simulink model "Boeing787_debug"  (R2013a)
settings: Solver=ode23tb  SolverMode=SingleTasking  StartTime=0.0  StopTime=18000  RelTol=1e-3
InitFcn:
  | load('SampleOutput.mat')
  | 
  | load('SampleFuelBurn.mat')
StartFcn:
  | tic
StopFcn:
  | ttt = toc
  | tend = eval(get_param(bdroot,'StopTime'));
  | disp(['Total Simulation Time (s) = ' num2str(ttt) 's']);
  | RTR =  ttt/tend
  | disp(['Simulation Speed is ' num2str(tend/ttt) 'x faster than real-time']);
values from neighbouring files (symbols this model uses):
  FuelBurn = [0 0 0 0 0 0 0 0 0 0 0 0 ... (18249 elements, 1x18249)]    [Benchmark_data1.mat]
undefined symbols (not defined in the file or in its folder): CurrentMission, seed
libraries: PowerFlowLib x20, simulink x14, powerlib_meascontrol x3
(part 15 of 17)

== system Boeing787_debug/Electrical/Generation Unit Sync-Sync5/Generator ==
  note: Dynamic model of P.U. Synchronous Generators v1.0
      | Base frequency is 60 Hz
      | Network transients are omitted
      | by Tutku Buyukdegirmenci
  note: Core Dynaimcs
  note: Outputs
  note: Inputs
  note: 0 axis to be implemented
  idq0 : Inport
  w : Inport  Port=2
  ifd' : Inport  Port=3
  Temp : Inport  Port=4
  Demux : Demux  Outputs=3
  Divide : Product  Inputs=*/
  Dynamics : Subsystem
  Electromagnetic Torque Output Power : Subsystem
  Gain1 : Gain  Gain=Xmd/R_fd/VBFD
  Gain2 : Gain  Gain=1/wB
  Gain3 : Gain  Gain=R_fd*VBFD/IBFD
  Gain4 : Gain  Gain=P/2
  Generator Power Loss : Subsystem
  Mux : Mux  Inputs=3
  Product : Product
  Stator Voltage : Subsystem
  Terminator2 : Terminator
  Terminator3 : Terminator
  Terminator4 : Terminator
  V0 : Constant  Value=0
  p.u. transform currents : Gain  Gain=-1/IBDQ
  p.u. transform torque : Gain  Gain=TB
  p.u. transform voltages : Gain  Gain=VBDQ
  vdq0 : Outport
  Te : Outport  Port=2
  vfd' : Outport  Port=3
  Ploss : Outport  Port=4
  wires:
  Gain4/1 -> Gain2/1
  [Efd] -> Dynamics/3(Efd)
  ifd'/1 -> Gain3/1
  idq0/1 -> p.u. transform currents/1
  p.u. transform voltages/1 -> vdq0/1
  Generator Power Loss/3(PLOSS) -> Ploss/1, Terminator4/1
  Generator Power Loss/2(PM) -> Terminator3/1
  Generator Power Loss/1(PE) -> Terminator2/1
  [Te] -> Generator Power Loss/5(Te)
  [nu] -> Generator Power Loss/6(w/ws)
  [Iq] -> Generator Power Loss/4(Iq)
  [Id] -> Generator Power Loss/3(Id)
  [Vq] -> Generator Power Loss/2(Eq)
  [Vd] -> Generator Power Loss/1(Ed)
  p.u. transform torque/1 -> Te/1
  p.u. transform currents/1 -> Demux/1
  [Te] -> p.u. transform torque/1
  Electromagnetic Torque Output Power/1(TE) -> [Te]
  [nu] -> Stator Voltage/7(w/ws)
  V0/1 -> Mux/3
  [Vq] -> Mux/2
  [Vd] -> Mux/1
  Mux/1 -> p.u. transform voltages/1
  [Iq] -> Electromagnetic Torque Output Power/2(Iq), Stator Voltage/2(Iq)
  [Id] -> Electromagnetic Torque Output Power/1(Id), Stator Voltage/1(Id)
  [Iq] -> Dynamics/2(Iq)
  [Id] -> Dynamics/1(Id)
  Gain2/1 -> [nu]
  Demux/2 -> [Iq]
  Demux/1 -> [Id]
  w/1 -> Gain4/1
  Stator Voltage/1(Ed) -> [Vd]
  Stator Voltage/2(Eq) -> [Vq]
  Dynamics/4(Phi_2q) -> Electromagnetic Torque Output Power/6(Phi_2q), Stator Voltage/6(Phi_2q)
  Dynamics/3(Phi_1d) -> Electromagnetic Torque Output Power/5(Phi_1d), Stator Voltage/5(Phi_1d)
  Dynamics/2(Ed1) -> Electromagnetic Torque Output Power/4(Ed1), Stator Voltage/4(Ed1)
  Dynamics/1(Eq1) -> Electromagnetic Torque Output Power/3(Eq1), Stator Voltage/3(Eq1)
  Temp/1 -> [R_temp_delta]
  Gain1/1 -> Divide/1
  Divide/1 -> [Efd]
  Gain3/1 -> Product/1  "vfd'"
  Product/1 -> Gain1/1, vfd'/1
  [R_temp_delta] -> Divide/2, Product/2
  [R_temp_delta] -> Stator Voltage/8(Temp), Dynamics/4(Temp)

== system Boeing787_debug/Electrical/Thermal Interface/Battery Thermal Model ==
  Ploss : Inport
  Liquid Coolant Temp : Inport  Port=2
  Air Temp : Inport  Port=3
  coolant mdot : Inport  Port=4
  Integrator : Integrator  InitialCondition=20
  MATLAB Function : MATLAB Function  TreatAsAtomicUnit=on
  T_Batt : Outport
  wires:
  Ploss/1 -> MATLAB Function/1(Ploss)
  Liquid Coolant Temp/1 -> MATLAB Function/2(Tf)
  MATLAB Function/1(Tdot) -> Integrator/1
  Integrator/1 -> MATLAB Function/5(Tgen), T_Batt/1
  coolant mdot/1 -> MATLAB Function/4(mdot_f)
  Air Temp/1 -> MATLAB Function/3(Ta)

== system Boeing787_debug/Electrical/Thermal Interface/Generator 1 Thermal Model ==
  Ploss : Inport
  Liquid Coolant Temp : Inport  Port=2
  Air Temp : Inport  Port=3
  coolant mdot : Inport  Port=4
  Integrator : Integrator  InitialCondition=20
  MATLAB Function : MATLAB Function  TreatAsAtomicUnit=on
  T_gen : Outport
  wires:
  Ploss/1 -> MATLAB Function/1(Ploss)
  Liquid Coolant Temp/1 -> MATLAB Function/2(Tf)
  MATLAB Function/1(Tdot) -> Integrator/1
  Integrator/1 -> MATLAB Function/5(Tgen), T_gen/1
  coolant mdot/1 -> MATLAB Function/4(mdot_f)
  Air Temp/1 -> MATLAB Function/3(Ta)

== system Boeing787_debug/Electrical/Thermal Interface/Generator 2 Thermal Model ==
  Ploss : Inport
  Liquid Coolant Temp : Inport  Port=2
  Air Temp : Inport  Port=3
  coolant mdot : Inport  Port=4
  Integrator : Integrator  InitialCondition=20
  MATLAB Function : MATLAB Function  TreatAsAtomicUnit=on
  T_gen : Outport
  wires:
  Air Temp/1 -> MATLAB Function/3(Ta)
  coolant mdot/1 -> MATLAB Function/4(mdot_f)
  Integrator/1 -> T_gen/1, MATLAB Function/5(Tgen)
  MATLAB Function/1(Tdot) -> Integrator/1
  Liquid Coolant Temp/1 -> MATLAB Function/2(Tf)
  Ploss/1 -> MATLAB Function/1(Ploss)

== system Boeing787_debug/Electrical/Thermal Interface/Generator 3 Thermal Model ==
  Ploss : Inport
  Liquid Coolant Temp : Inport  Port=2
  Air Temp : Inport  Port=3
  coolant mdot : Inport  Port=4
  Integrator : Integrator  InitialCondition=20
  MATLAB Function : MATLAB Function  TreatAsAtomicUnit=on
  T_gen : Outport
  wires:
  Ploss/1 -> MATLAB Function/1(Ploss)
  Liquid Coolant Temp/1 -> MATLAB Function/2(Tf)
  MATLAB Function/1(Tdot) -> Integrator/1
  Integrator/1 -> MATLAB Function/5(Tgen), T_gen/1
  coolant mdot/1 -> MATLAB Function/4(mdot_f)
  Air Temp/1 -> MATLAB Function/3(Ta)

== system Boeing787_debug/Electrical/Thermal Interface/Generator 4 Thermal Model ==
  Ploss : Inport
  Liquid Coolant Temp : Inport  Port=2
  Air Temp : Inport  Port=3
  coolant mdot : Inport  Port=4
  Integrator : Integrator  InitialCondition=20
  MATLAB Function : MATLAB Function  TreatAsAtomicUnit=on
  T_gen : Outport
  wires:
  Air Temp/1 -> MATLAB Function/3(Ta)
  coolant mdot/1 -> MATLAB Function/4(mdot_f)
  Integrator/1 -> T_gen/1, MATLAB Function/5(Tgen)
  MATLAB Function/1(Tdot) -> Integrator/1
  Liquid Coolant Temp/1 -> MATLAB Function/2(Tf)
  Ploss/1 -> MATLAB Function/1(Ploss)

== system Boeing787_debug/Electrical/Thermal Interface/Generator 5 Thermal Model ==
  Ploss : Inport
  Liquid Coolant Temp : Inport  Port=2
  Air Temp : Inport  Port=3
  coolant mdot : Inport  Port=4
  Integrator : Integrator  InitialCondition=20
  MATLAB Function : MATLAB Function  TreatAsAtomicUnit=on
  T_gen : Outport
  wires:
  Ploss/1 -> MATLAB Function/1(Ploss)
  Liquid Coolant Temp/1 -> MATLAB Function/2(Tf)
  MATLAB Function/1(Tdot) -> Integrator/1
  Integrator/1 -> MATLAB Function/5(Tgen), T_gen/1
  coolant mdot/1 -> MATLAB Function/4(mdot_f)
  Air Temp/1 -> MATLAB Function/3(Ta)

== system Boeing787_debug/Electrical/Thermal Interface/Generator 6 Thermal Model ==
  Ploss : Inport
  Liquid Coolant Temp : Inport  Port=2
  Air Temp : Inport  Port=3
  coolant mdot : Inport  Port=4
  Integrator : Integrator  InitialCondition=20
  MATLAB Function : MATLAB Function  TreatAsAtomicUnit=on
  T_gen : Outport
  wires:
  Air Temp/1 -> MATLAB Function/3(Ta)
  coolant mdot/1 -> MATLAB Function/4(mdot_f)
  Integrator/1 -> T_gen/1, MATLAB Function/5(Tgen)
  MATLAB Function/1(Tdot) -> Integrator/1
  Liquid Coolant Temp/1 -> MATLAB Function/2(Tf)
  Ploss/1 -> MATLAB Function/1(Ploss)

== system Boeing787_debug/Electrical/Thermal Interface/Load Thermal Model ==
  Ploss : Inport
  Liquid Coolant Temp : Inport  Port=2
  Air Temp : Inport  Port=3
  coolant mdot : Inport  Port=4
  Integrator : Integrator  InitialCondition=20
  MATLAB Function : MATLAB Function  TreatAsAtomicUnit=on
  T_gen : Outport
  wires:
  Air Temp/1 -> MATLAB Function/3(Ta)
  coolant mdot/1 -> MATLAB Function/4(mdot_f)
  Integrator/1 -> T_gen/1, MATLAB Function/5(Tgen)
  MATLAB Function/1(Tdot) -> Integrator/1
  Liquid Coolant Temp/1 -> MATLAB Function/2(Tf)
  Ploss/1 -> MATLAB Function/1(Ploss)

== system Boeing787_debug/Electrical/Transformer-rectifier/Control New ==
  Vout : Inport
  ref : Inport  Port=2
  Gain1 : Gain
  Integrator1 : Integrator  ExternalReset=rising
  Ki1 : Gain  Gain=10
  Kp e(t)1 : Gain  Gain=10
  PID Controller : simulink/Continuous/PID Controller  Controller=PID  TimeDomain=Continuous-time  SampleTime=1  IntegratorMethod=Forward Euler  FilterMethod=Forward Euler  Form=Parallel  P=0  I=-20.0000452359282  D=0  N=100  InitialConditionSource=internal  InitialConditionForIntegrator=0  InitialConditionForFilter=0  ExternalReset=none  LimitOutput=off  UpperSaturationLimit=inf  LowerSaturationLimit=-inf  LinearizeAsGain=on  AntiWindupMode=none  Kb=1  TrackingMode=off  Kt=1  PParamMin=[]  PParamMax=[]  IParamMin=[]  IParamMax=[]  DParamMin=[]  DParamMax=[]  NParamMin=[]  NParamMax=[]  KbParamMin=[]  KbParamMax=[]  KtParamMin=[]  KtParamMax=[]  POutMin=[]  POutMax=[]  IOutMin=[]  IOutMax=[]  DOutMin=[]  DOutMax=[]  NOutMin=[]  NOutMax=[]  KbOutMin=[]  KbOutMax=[]  KtOutMin=[]  KtOutMax=[]  IntegratorOutMin=[]  IntegratorOutMax=[]  FilterOutMin=[]  FilterOutMax=[]  SumOutMin=[]  SumOutMax=[]  SumI1OutMin=[]  SumI1OutMax=[]  SumI2OutMin=[]  SumI2OutMax=[]  SumI3OutMin=[]  SumI3OutMax=[]  SumDOutMin=[]  SumDOutMax=[]  SaturationOutMin=[]  SaturationOutMax=[]  IntegratorContinuousStateAttributes=''  IntegratorStateMustResolveToSignalObject=off  IntegratorRTWStateStorageClass=Auto  FilterContinuousStateAttributes=''  FilterStateMustResolveToSignalObject=off  FilterRTWStateStorageClass=Auto
  Reset on controller start1 : Step  Time=75  SampleTime=0
  Sum : Sum  Inputs=|-+
  Sum2 : Sum  Inputs=|++
  u : Outport
  wires:
  Sum/1 -> PID Controller/1
  Integrator1/1 -> Sum2/1
  Kp e(t)1/1 -> Sum2/2
  Ki1/1 -> Integrator1/1
  Reset on controller start1/1 -> Integrator1/2
  ? -> Kp e(t)1/1, Ki1/1
  Gain1/1 -> u/1
  ref/1 -> Sum/2
  Vout/1 -> Sum/1
  PID Controller/1 -> Gain1/1

== system Boeing787_debug/Electrical/Transformer-rectifier/Control old ==
  Vout : Inport
  ref : Inport  Port=2
  Clock : Clock
  Constant2 : Constant  Value=0
  Dead Zone : DeadZone  LowerValue=-2  UpperValue=2  SaturateOnIntegerOverflow=on
  Gain : Gain
  Gain1 : Gain  Gain=-1
  Integrator : Integrator  ExternalReset=rising
  MinMax : MinMax  Function=max
  Reset on controller start : Step  Time=75  SampleTime=0
  Sum : Sum  Inputs=|-+
  Switch : Switch  Criteria=u2 > Threshold  Threshold=75
  u : Outport
  wires:
  Vout/1 -> MinMax/1
  Dead Zone/1 -> Gain/1
  Gain1/1 -> u/1
  Gain/1 -> Integrator/1
  ref/1 -> Sum/2
  Clock/1 -> Switch/2
  Constant2/1 -> Switch/3
  MinMax/1 -> Sum/1
  Switch/1 -> Gain1/1
  Reset on controller start/1 -> Integrator/2
  Sum/1 -> Dead Zone/1
  Integrator/1 -> Switch/1

== system Boeing787_debug/Electrical/Transformer-rectifier/Three-phase Full Bridge Rectifier ==
  iout : Inport
  vin : Inport  Port=2
  u : Inport  Port=3
  1/C : Gain  Gain=1/C  SaturateOnIntegerOverflow=on  OutDataTypeStr=Inherit: Same as input  ParamDataTypeStr=Inherit: Same as input
  1/Rc : Gain  Gain=1/Rc  SaturateOnIntegerOverflow=on  OutDataTypeStr=Inherit: Same as input  ParamDataTypeStr=Inherit: Same as input
  Abs : Abs  SaturateOnIntegerOverflow=on
  Constant : Constant
  Constant1 : Constant  Value=800*pi
  Demux : Demux  Outputs=3
  Demux1 : Demux  Outputs=3
  Integrator : Integrator
  MinMax1 : MinMax  Function=max
  Mux : Mux  Inputs=3
  Mux1 : Mux  Inputs=3
  Product : Product  RndMeth=Zero
  Saturation : Saturate  UpperLimit=inf  LowerLimit=0
  Sum{,1..7} (8 alike) : Sum  Inputs=+-  SaturateOnIntegerOverflow=on  InputSameDT=on  OutDataTypeStr=Inherit: Same as first input
  Sum8 : Sum  Inputs=|++
  dq0 to abc : powerlib_meascontrol/Transformations/dq0 to abc  Alignment=90 degrees behind phase A axis
  vout : Outport
  iin : Outport  Port=2
  wires:
  Saturation/1 -> Sum1/1, Product/2
  1/C/1 -> Integrator/1
  Sum1/1 -> 1/C/1
  Integrator/1 -> Sum8/1, vout/1
  1/Rc/1 -> Saturation/1
  iout/1 -> Sum1/2
  Sum/1 -> 1/Rc/1
  Product/1 -> iin/1
  MinMax1/1 -> Sum/1
  Abs/1 -> MinMax1/1
  u/1 -> Sum8/2
  Sum8/1 -> Sum/2
  Constant/1 -> Product/1
  ? -> Demux1/1
  Mux1/1 -> ?
  Demux1/1 -> Sum7/2, Sum5/1
  Demux1/2 -> Sum5/2, Sum6/1
  Demux1/3 -> Sum7/1, Sum6/2
  Sum5/1 -> Mux1/1
  Sum6/1 -> Mux1/2
  Sum7/1 -> Mux1/3
  Sum4/1 -> Mux/3
  Sum3/1 -> Mux/2
  Sum2/1 -> Mux/1
  Demux/3 -> Sum3/2, Sum4/1
  Demux/2 -> Sum3/1, Sum2/2
  Demux/1 -> Sum2/1, Sum4/2
  Mux/1 -> Abs/1
  vin/1 -> dq0 to abc/1
  dq0 to abc/1 -> Demux/1
  Constant1/1 -> dq0 to abc/2

== system Boeing787_debug/Electrical/Transformer-rectifier/Transformer1 ==
  Vin : Inport
  Iout : Inport  Port=2
  Gain : Gain  Gain=N2/N1
  Gain1 : Gain  Gain=N2/N1
  Gain2 : Gain  Gain=Rp
  Gain3 : Gain  Gain=Rs
  Scope : Scope
      settings: YMin=-28.76938  YMax=258.92445  SaveName=ScopeData11
  Sum1 : Sum  Inputs=|+-
  Sum2 : Sum  Inputs=|+-
  Vout : Outport
  Iin : Outport  Port=2
  wires:
  Gain3/1 -> Sum2/2
  Gain1/1 -> Iin/1, Gain2/1
  Sum2/1 -> Vout/1
  Gain/1 -> Sum2/1
  Sum1/1 -> Gain/1
  Gain2/1 -> Sum1/2
  Vin/1 -> Sum1/1
  Iout/1 -> Scope/1, Gain3/1, Gain1/1

== system Boeing787_debug/Electrical/Transformer-rectifier1/Control New ==
  Vout : Inport
  ref : Inport  Port=2
  Gain1 : Gain
  Integrator1 : Integrator  ExternalReset=rising
  Ki1 : Gain  Gain=10
  Kp e(t)1 : Gain  Gain=10
  PID Controller : simulink/Continuous/PID Controller  Controller=PID  TimeDomain=Continuous-time  SampleTime=1  IntegratorMethod=Forward Euler  FilterMethod=Forward Euler  Form=Parallel  P=0  I=-20.0000452359282  D=0  N=100  InitialConditionSource=internal  InitialConditionForIntegrator=0  InitialConditionForFilter=0  ExternalReset=none  LimitOutput=off  UpperSaturationLimit=inf  LowerSaturationLimit=-inf  LinearizeAsGain=on  AntiWindupMode=none  Kb=1  TrackingMode=off  Kt=1  PParamMin=[]  PParamMax=[]  IParamMin=[]  IParamMax=[]  DParamMin=[]  DParamMax=[]  NParamMin=[]  NParamMax=[]  KbParamMin=[]  KbParamMax=[]  KtParamMin=[]  KtParamMax=[]  POutMin=[]  POutMax=[]  IOutMin=[]  IOutMax=[]  DOutMin=[]  DOutMax=[]  NOutMin=[]  NOutMax=[]  KbOutMin=[]  KbOutMax=[]  KtOutMin=[]  KtOutMax=[]  IntegratorOutMin=[]  IntegratorOutMax=[]  FilterOutMin=[]  FilterOutMax=[]  SumOutMin=[]  SumOutMax=[]  SumI1OutMin=[]  SumI1OutMax=[]  SumI2OutMin=[]  SumI2OutMax=[]  SumI3OutMin=[]  SumI3OutMax=[]  SumDOutMin=[]  SumDOutMax=[]  SaturationOutMin=[]  SaturationOutMax=[]  IntegratorContinuousStateAttributes=''  IntegratorStateMustResolveToSignalObject=off  IntegratorRTWStateStorageClass=Auto  FilterContinuousStateAttributes=''  FilterStateMustResolveToSignalObject=off  FilterRTWStateStorageClass=Auto
  Reset on controller start1 : Step  Time=75  SampleTime=0
  Sum : Sum  Inputs=|-+
  Sum2 : Sum  Inputs=|++
  u : Outport
  wires:
  Sum/1 -> PID Controller/1
  Integrator1/1 -> Sum2/1
  Kp e(t)1/1 -> Sum2/2
  Ki1/1 -> Integrator1/1
  Reset on controller start1/1 -> Integrator1/2
  ? -> Kp e(t)1/1, Ki1/1
  Gain1/1 -> u/1
  ref/1 -> Sum/2
  Vout/1 -> Sum/1
  PID Controller/1 -> Gain1/1

== system Boeing787_debug/Electrical/Transformer-rectifier1/Control old ==
  Vout : Inport
  ref : Inport  Port=2
  Clock : Clock
  Constant2 : Constant  Value=0
  Gain1 : Gain  Gain=-1
  Integrator : Integrator  ExternalReset=rising
  Ki : Gain  Gain=10
  Kp e(t) : Gain  Gain=10
  MinMax : MinMax  Function=max
  Reset on controller start : Step  Time=75  SampleTime=0
  Sum : Sum  Inputs=|-+
  Sum1 : Sum  Inputs=|++
  Switch : Switch  Criteria=u2 > Threshold  Threshold=75
  u : Outport
  wires:
  Vout/1 -> MinMax/1
  Sum/1 -> Kp e(t)/1, Ki/1
  Reset on controller start/1 -> Integrator/2
  Switch/1 -> Gain1/1
  MinMax/1 -> Sum/1
  Constant2/1 -> Switch/3
  Clock/1 -> Switch/2
  ref/1 -> Sum/2
  Ki/1 -> Integrator/1
  Gain1/1 -> u/1
  Kp e(t)/1 -> Sum1/2
  Integrator/1 -> Sum1/1
  Sum1/1 -> Switch/1

== system Boeing787_debug/Electrical/Transformer-rectifier1/Three-phase Full Bridge1 ==
  iout : Inport
  vin : Inport  Port=2
  u : Inport  Port=3
  vin1 : Inport  Port=4
  1/C : Gain  Gain=1/C  SaturateOnIntegerOverflow=on  OutDataTypeStr=Inherit: Same as input  ParamDataTypeStr=Inherit: Same as input
  1/Rc : Gain  Gain=1/Rc  SaturateOnIntegerOverflow=on  OutDataTypeStr=Inherit: Same as input  ParamDataTypeStr=Inherit: Same as input
  Abs : Abs  SaturateOnIntegerOverflow=on
  Constant : Constant  Value=800*pi
  Demux : Demux  Outputs=3
  Demux1 : Demux  Outputs=3
  Integrator : Integrator
  MinMax1 : MinMax  Function=max
  Mux : Mux  Inputs=3
  Mux1 : Mux  Inputs=3
  Saturation : Saturate  UpperLimit=inf  LowerLimit=0
  Scope : Scope
      settings: YMin=-3.32249  YMax=29.90241  SaveName=ScopeData12
  Sum{,1..4,6..8} (8 alike) : Sum  Inputs=+-  SaturateOnIntegerOverflow=on  InputSameDT=on  OutDataTypeStr=Inherit: Same as first input
  Sum5 : Sum  SaturateOnIntegerOverflow=on  InputSameDT=on  OutDataTypeStr=Inherit: Same as first input
  dq0 to abc : powerlib_meascontrol/Transformations/dq0 to abc  Alignment=90 degrees behind phase A axis
  vout : Outport
  iin : Outport  Port=2
  wires:
  Sum5/1 -> Sum/2
  u/1 -> Sum5/2
  Abs/1 -> MinMax1/1
  MinMax1/1 -> Sum/1
  Saturation/1 -> iin/1, Scope/1, Sum1/1
  Sum/1 -> 1/Rc/1
  iout/1 -> Sum1/2
  1/Rc/1 -> Saturation/1
  Integrator/1 -> Sum5/1, vout/1
  Sum1/1 -> 1/C/1
  1/C/1 -> Integrator/1
  Sum8/1 -> Mux1/3
  Sum7/1 -> Mux1/2
  Sum6/1 -> Mux1/1
  Demux1/3 -> Sum7/2, Sum8/1
  Demux1/2 -> Sum7/1, Sum6/2
  Demux1/1 -> Sum6/1, Sum8/2
  Mux1/1 -> ?
  vin1/1 -> Demux1/1
  Sum4/1 -> Mux/3
  Sum3/1 -> Mux/2
  Sum2/1 -> Mux/1
  Demux/3 -> Sum3/2, Sum4/1
  Demux/2 -> Sum3/1, Sum2/2
  Demux/1 -> Sum2/1, Sum4/2
  Mux/1 -> Abs/1
  dq0 to abc/1 -> Demux/1
  vin/1 -> dq0 to abc/1
  Constant/1 -> dq0 to abc/2

== system Boeing787_debug/Electrical/Transformer-rectifier1/Transformer1 ==
  Vin : Inport
  Iout : Inport  Port=2
  Gain : Gain  Gain=N2/N1
  Gain1 : Gain  Gain=N2/N1
  Gain2 : Gain  Gain=Rp
  Gain3 : Gain  Gain=Rs
  Memory1 : Memory
  Scope : Scope
      settings: YMin=-1.03024  YMax=9.27213  SaveName=ScopeData11
  Sum1 : Sum  Inputs=|+-
  Sum2 : Sum  Inputs=|+-
  Vout : Outport
  Iin : Outport  Port=2
  wires:
  Memory1/1 -> Gain1/1, Gain3/1, Scope/1
  Iout/1 -> Memory1/1
  Vin/1 -> Sum1/1
  Gain2/1 -> Sum1/2
  Sum1/1 -> Gain/1
  Gain/1 -> Sum2/1
  Sum2/1 -> Vout/1
  Gain1/1 -> Gain2/1, Iin/1
  Gain3/1 -> Sum2/2

== system Boeing787_debug/Electrical/Enabled_AC_Loadloss/Enabled Subsystem/CURRENT BASED LOADS ==
  note: SPLITTING CURRENT IN BOTH D AND Q AXES
  Constant : Constant  Value=0
  Constant1 : Constant  Value=ILRMS
  Gain1 : Gain  Gain=sqrt(2)
  Mux : Mux  Inputs=3
  Idqo : Outport
  wires:
  Constant/1 -> Mux/3
  Mux/1 -> Idqo/1
  Gain1/1 -> Mux/2, Mux/1
  Constant1/1 -> Gain1/1

== system Boeing787_debug/Electrical/Enabled_AC_Loadloss/Enabled Subsystem/IMPEDANCE BASED LOADS ==
  Vdq0 : Inport
  Constant1 : Constant  Value=R
  Constant2 : Constant  Value=X
  Constant3 : Constant  Value=R
  Constant4 : Constant  Value=X
  Demux : Demux  Outputs=3
  Fcn : Fcn  Expr=u(1)/(u(2)+0.1)
  Fcn1 : Fcn  Expr=u(1)/(u(2)+0.1)
  Math Function{,1..3} (4 alike) : Math  Operator=square  SaturateOnIntegerOverflow=on
  Mux : Mux  Inputs=3
  Mux1 : Mux  Inputs=2
  Mux2 : Mux  Inputs=2
  Product{1..2,5..6} (4 alike) : Product  Inputs=**  RndMeth=Zero
  Sum1 : Sum  Inputs=|++
  Sum2 : Sum  Inputs=|++
  Sum3 : Sum  Inputs=|+-
  Sum4 : Sum  Inputs=|++
  Idq0 : Outport
  wires:
  Fcn1/1 -> Mux/2
  Fcn/1 -> Mux/1
  Vdq0/1 -> Demux/1
  Constant1/1 -> Product1/1, Math Function/1
  Demux/1 -> Product1/2, Product6/2
  Product1/1 -> Sum1/1
  Demux/2 -> Product2/2, Product5/2
  Constant2/1 -> Product2/1, Math Function1/1
  Product2/1 -> Sum1/2
  Sum1/1 -> Mux1/1
  Math Function/1 -> Sum2/1
  Math Function1/1 -> Sum2/2
  Sum2/1 -> Mux1/2
  Constant3/1 -> Product5/1, Math Function2/1
  Product5/1 -> Sum3/1
  Constant4/1 -> Product6/1, Math Function3/1
  Product6/1 -> Sum3/2
  Math Function2/1 -> Sum4/1
  Math Function3/1 -> Sum4/2
  Sum3/1 -> Mux2/1
  Sum4/1 -> Mux2/2
  Mux1/1 -> Fcn/1
  Mux2/1 -> Fcn1/1
  Mux/1 -> Idq0/1

== system Boeing787_debug/Electrical/Enabled_AC_Loadloss/Enabled Subsystem/POWER BASED LOADS ==
  Vdq0 : Inport
  Constant1 : Constant  Value=P
  Constant2 : Constant  Value=PF
  Constant3 : Constant  Value=P
  Constant5 : Constant
  Constant6 : Constant  Value=0
  Constant7 : Constant  Value=P
  Demux : Demux  Outputs=3
  Fcn : Fcn  Expr=u(1)/(u(2)+0.1)
  Fcn1 : Fcn  Expr=u(1)/(u(2)+0.1)
  Math Function{,1..3} (4 alike) : Math  Operator=square  SaturateOnIntegerOverflow=on
  Mux : Mux  Inputs=3
  Mux1 : Mux  Inputs=2
  Mux2 : Mux  Inputs=2
  Product1 : Product  Inputs=***  RndMeth=Zero
  Product2 : Product  Inputs=**  RndMeth=Zero
  Product3 : Product  Inputs=**  RndMeth=Zero
  Product5 : Product  Inputs=***  RndMeth=Zero
  Product6 : Product  Inputs=**  RndMeth=Zero
  Sum1 : Sum  Inputs=|++
  Sum2 : Sum  Inputs=|++
  Sum3 : Sum  Inputs=|+-
  Sum4 : Sum  Inputs=|++
  Trigonometric Function : Trigonometry  Operator=acos
  Trigonometric Function1 : Trigonometry  Operator=tan
  Idq0 : Outport
  loss : Outport  Port=2
  wires:
  Constant1/1 -> Product1/1, loss/1
  Constant6/1 -> Product5/3
  Constant5/1 -> Product1/3
  Mux/1 -> Idq0/1
  Mux2/1 -> Fcn1/1
  Mux1/1 -> Fcn/1
  Sum4/1 -> Mux2/2
  Sum3/1 -> Mux2/1
  Math Function3/1 -> Sum4/2
  Math Function2/1 -> Sum4/1
  Product6/1 -> Sum3/2
  Product3/1 -> Product6/1, Product2/1
  Product5/1 -> Sum3/1
  Constant3/1 -> Product5/1
  Sum2/1 -> Mux1/2
  Math Function1/1 -> Sum2/2
  Math Function/1 -> Sum2/1
  Sum1/1 -> Mux1/1
  Product2/1 -> Sum1/2
  Constant2/1 -> Trigonometric Function/1
  Demux/2 -> Math Function2/1, Product5/2, Math Function1/1, Product2/2
  Product1/1 -> Sum1/1
  Demux/1 -> Math Function3/1, Product6/2, Math Function/1, Product1/2
  Vdq0/1 -> Demux/1
  Fcn/1 -> Mux/1
  Fcn1/1 -> Mux/2
  Trigonometric Function/1 -> Trigonometric Function1/1
  Trigonometric Function1/1 -> Product3/1
  Constant7/1 -> Product3/2

== system Boeing787_debug/Electrical/Enabled_AC_Loadloss/Enabled Subsystem1/CURRENT BASED LOADS ==
  note: SPLITTING CURRENT IN BOTH D AND Q AXES
  Iconst RMS : Inport
  Gain1 : Gain  Gain=sqrt(2)
  Mux : Mux  Inputs=3
  Idqo : Outport
  wires:
  Iconst RMS/1 -> Gain1/1
  Gain1/1 -> Mux/1, Mux/2
  Mux/1 -> Idqo/1

== system Boeing787_debug/Electrical/Enabled_AC_Loadloss/Enabled Subsystem1/POWER BASED LOADS ==
  Vdq0 : Inport
  P : Inport  Port=2
  Q : Inport  Port=3
  Demux : Demux  Outputs=3
  Fcn : Fcn  Expr=u(1)/(u(2)+0.1)
  Fcn1 : Fcn  Expr=u(1)/(u(2)+0.1)
  Math Function{,1..3} (4 alike) : Math  Operator=square  SaturateOnIntegerOverflow=on
  Mux : Mux  Inputs=3
  Mux1 : Mux  Inputs=2
  Mux2 : Mux  Inputs=2
  Product{1..2,5..6} (4 alike) : Product  Inputs=**  RndMeth=Zero
  Sum1 : Sum  Inputs=|++
  Sum2 : Sum  Inputs=|++
  Sum3 : Sum  Inputs=|+-
  Sum4 : Sum  Inputs=|++
  Idq0 : Outport
  wires:
  Demux/1 -> Math Function/1, Product1/2, Product6/2, Math Function3/1
  Vdq0/1 -> Demux/1
  P/1 -> Product1/1, Product5/1
  Product1/1 -> Sum1/1
  Demux/2 -> Product2/2, Math Function1/1, Product5/2, Math Function2/1
  Q/1 -> Product2/1, Product6/1
  Product2/1 -> Sum1/2
  Sum1/1 -> Mux1/1
  Math Function/1 -> Sum2/1
  Math Function1/1 -> Sum2/2
  Sum2/1 -> Mux1/2
  Product5/1 -> Sum3/1
  Product6/1 -> Sum3/2
  Math Function2/1 -> Sum4/1
  Math Function3/1 -> Sum4/2
  Sum3/1 -> Mux2/1
  Sum4/1 -> Mux2/2
  Mux1/1 -> Fcn/1
  Mux2/1 -> Fcn1/1
  Mux/1 -> Idq0/1
  Fcn/1 -> Mux/1
  Fcn1/1 -> Mux/2

== system Boeing787_debug/Electrical/Enabled_AC_Loadloss1/Enabled Subsystem/CURRENT BASED LOADS ==
  note: SPLITTING CURRENT IN BOTH D AND Q AXES
  Constant : Constant  Value=0
  Constant1 : Constant  Value=ILRMS
  Gain1 : Gain  Gain=sqrt(2)
  Mux : Mux  Inputs=3
  Idqo : Outport
  wires:
  Constant/1 -> Mux/3
  Mux/1 -> Idqo/1
  Gain1/1 -> Mux/2, Mux/1
  Constant1/1 -> Gain1/1

== system Boeing787_debug/Electrical/Enabled_AC_Loadloss1/Enabled Subsystem/IMPEDANCE BASED LOADS ==
  Vdq0 : Inport
  Constant1 : Constant  Value=R
  Constant2 : Constant  Value=X
  Constant3 : Constant  Value=R
  Constant4 : Constant  Value=X
  Demux : Demux  Outputs=3
  Fcn : Fcn  Expr=u(1)/(u(2)+0.1)
  Fcn1 : Fcn  Expr=u(1)/(u(2)+0.1)
  Math Function{,1..3} (4 alike) : Math  Operator=square  SaturateOnIntegerOverflow=on
  Mux : Mux  Inputs=3
  Mux1 : Mux  Inputs=2
  Mux2 : Mux  Inputs=2
  Product{1..2,5..6} (4 alike) : Product  Inputs=**  RndMeth=Zero
  Sum1 : Sum  Inputs=|++
  Sum2 : Sum  Inputs=|++
  Sum3 : Sum  Inputs=|+-
  Sum4 : Sum  Inputs=|++
  Transfer Fcn1 : TransferFcn  Denominator=[.01 1]
  Transfer Fcn2 : TransferFcn  Denominator=[.01 1]
  Idq0 : Outport
  wires:
  Fcn1/1 -> Transfer Fcn1/1
  Fcn/1 -> Transfer Fcn2/1
  Vdq0/1 -> Demux/1
  Constant1/1 -> Product1/1, Math Function/1
  Demux/1 -> Product1/2, Product6/2
  Product1/1 -> Sum1/1
  Demux/2 -> Product2/2, Product5/2
  Constant2/1 -> Product2/1, Math Function1/1
  Product2/1 -> Sum1/2
  Sum1/1 -> Mux1/1
  Math Function/1 -> Sum2/1
  Math Function1/1 -> Sum2/2
  Sum2/1 -> Mux1/2
  Constant3/1 -> Product5/1, Math Function2/1
  Product5/1 -> Sum3/1
  Constant4/1 -> Product6/1, Math Function3/1
  Product6/1 -> Sum3/2
  Math Function2/1 -> Sum4/1
  Math Function3/1 -> Sum4/2
  Sum3/1 -> Mux2/1
  Sum4/1 -> Mux2/2
  Mux1/1 -> Fcn/1
  Mux2/1 -> Fcn1/1
  Mux/1 -> Idq0/1
  Transfer Fcn2/1 -> Mux/1
  Transfer Fcn1/1 -> Mux/2

== system Boeing787_debug/Electrical/Enabled_AC_Loadloss1/Enabled Subsystem/POWER BASED LOADS ==
  Vdq0 : Inport
  Constant1 : Constant  Value=P
  Constant2 : Constant  Value=PF
  Constant3 : Constant  Value=P
  Constant5 : Constant
  Constant6 : Constant  Value=0
  Constant7 : Constant  Value=P
  Demux : Demux  Outputs=3
  Fcn : Fcn  Expr=u(1)/(u(2)+0.1)
  Fcn1 : Fcn  Expr=u(1)/(u(2)+0.1)
  Math Function{,1..3} (4 alike) : Math  Operator=square  SaturateOnIntegerOverflow=on
  Mux : Mux  Inputs=3
  Mux1 : Mux  Inputs=2
  Mux2 : Mux  Inputs=2
  Product1 : Product  Inputs=***  RndMeth=Zero
  Product2 : Product  Inputs=**  RndMeth=Zero
  Product3 : Product  Inputs=**  RndMeth=Zero
  Product5 : Product  Inputs=***  RndMeth=Zero
  Product6 : Product  Inputs=**  RndMeth=Zero
  Sum1 : Sum  Inputs=|++
  Sum2 : Sum  Inputs=|++
  Sum3 : Sum  Inputs=|+-
  Sum4 : Sum  Inputs=|++
  Transfer Fcn : TransferFcn  Denominator=[.01 1]
  Transfer Fcn1 : TransferFcn  Denominator=[.01 1]
  Transfer Fcn2 : TransferFcn  Denominator=[.01 1]
  Trigonometric Function : Trigonometry  Operator=acos
  Trigonometric Function1 : Trigonometry  Operator=tan
  Idq0 : Outport
  loss : Outport  Port=2
  wires:
  Constant1/1 -> Product1/1, Transfer Fcn2/1
  Constant6/1 -> Product5/3
  Constant5/1 -> Product1/3
  Mux/1 -> Idq0/1
  Mux2/1 -> Fcn1/1
  Mux1/1 -> Fcn/1
  Sum4/1 -> Mux2/2
  Sum3/1 -> Mux2/1
  Math Function3/1 -> Sum4/2
  Math Function2/1 -> Sum4/1
  Product6/1 -> Sum3/2
  Product3/1 -> Product6/1, Product2/1
  Product5/1 -> Sum3/1
  Constant3/1 -> Product5/1
  Sum2/1 -> Mux1/2
  Math Function1/1 -> Sum2/2
  Math Function/1 -> Sum2/1
  Sum1/1 -> Mux1/1
  Product2/1 -> Sum1/2
  Constant2/1 -> Trigonometric Function/1
  Demux/2 -> Math Function2/1, Product5/2, Math Function1/1, Product2/2
  Product1/1 -> Sum1/1
  Demux/1 -> Math Function3/1, Product6/2, Math Function/1, Product1/2
  Vdq0/1 -> Demux/1
  Fcn/1 -> Transfer Fcn/1
  Fcn1/1 -> Transfer Fcn1/1
  Trigonometric Function/1 -> Trigonometric Function1/1
  Trigonometric Function1/1 -> Product3/1
  Constant7/1 -> Product3/2
  Transfer Fcn/1 -> Mux/1
  Transfer Fcn1/1 -> Mux/2
  Transfer Fcn2/1 -> loss/1

== system Boeing787_debug/Electrical/Enabled_AC_Loadloss1/Enabled Subsystem1/CURRENT BASED LOADS ==
  note: SPLITTING CURRENT IN BOTH D AND Q AXES
  Iconst RMS : Inport
  Gain1 : Gain  Gain=sqrt(2)
  Mux : Mux  Inputs=3
  Idqo : Outport
  wires:
  Iconst RMS/1 -> Gain1/1
  Gain1/1 -> Mux/1, Mux/2
  Mux/1 -> Idqo/1

== system Boeing787_debug/Electrical/Enabled_AC_Loadloss1/Enabled Subsystem1/POWER BASED LOADS ==
  Vdq0 : Inport
  P : Inport  Port=2
  Q : Inport  Port=3
  Demux : Demux  Outputs=3
  Fcn : Fcn  Expr=u(1)/(u(2)+0.1)
  Fcn1 : Fcn  Expr=u(1)/(u(2)+0.1)
  Math Function{,1..3} (4 alike) : Math  Operator=square  SaturateOnIntegerOverflow=on
  Mux : Mux  Inputs=3
  Mux1 : Mux  Inputs=2
  Mux2 : Mux  Inputs=2
  Product{1..2,5..6} (4 alike) : Product  Inputs=**  RndMeth=Zero
  Sum1 : Sum  Inputs=|++
  Sum2 : Sum  Inputs=|++
  Sum3 : Sum  Inputs=|+-
  Sum4 : Sum  Inputs=|++
  Transfer Fcn1 : TransferFcn  Denominator=[.01 1]
  Transfer Fcn2 : TransferFcn  Denominator=[.01 1]
  Idq0 : Outport
  wires:
  Demux/1 -> Math Function/1, Product1/2, Product6/2, Math Function3/1
  Vdq0/1 -> Demux/1
  P/1 -> Product1/1, Product5/1
  Product1/1 -> Sum1/1
  Demux/2 -> Product2/2, Math Function1/1, Product5/2, Math Function2/1
  Q/1 -> Product2/1, Product6/1
  Product2/1 -> Sum1/2
  Sum1/1 -> Mux1/1
  Math Function/1 -> Sum2/1
  Math Function1/1 -> Sum2/2
  Sum2/1 -> Mux1/2
  Product5/1 -> Sum3/1
  Product6/1 -> Sum3/2
  Math Function2/1 -> Sum4/1
  Math Function3/1 -> Sum4/2
  Sum3/1 -> Mux2/1
  Sum4/1 -> Mux2/2
  Mux1/1 -> Fcn/1
  Mux2/1 -> Fcn1/1
  Mux/1 -> Idq0/1
  Fcn/1 -> Transfer Fcn2/1
  Fcn1/1 -> Transfer Fcn1/1
  Transfer Fcn2/1 -> Mux/1
  Transfer Fcn1/1 -> Mux/2

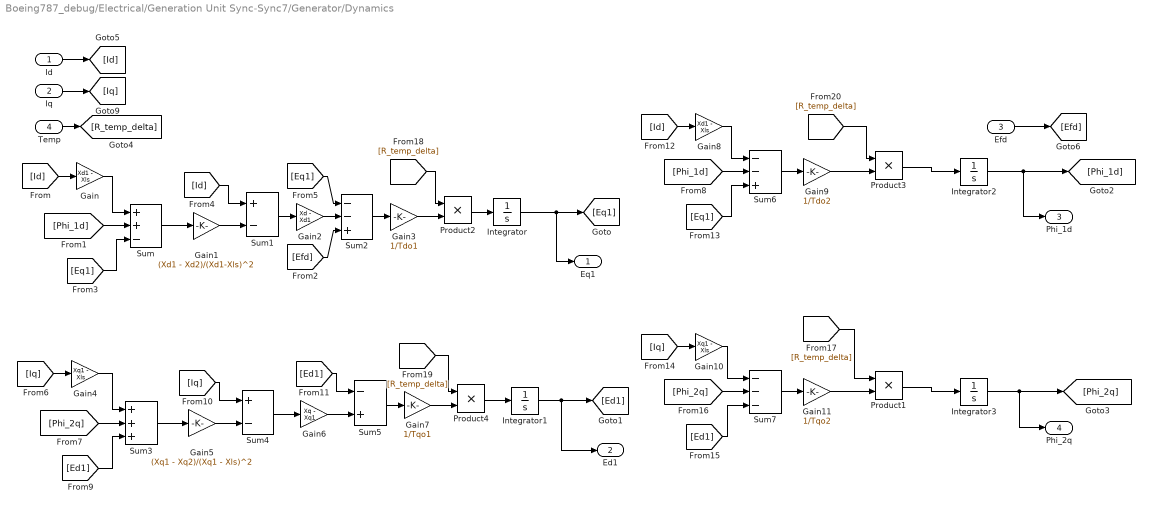
== system Boeing787_debug/Electrical/Generation Unit Sync-Sync7/Generator/Dynamics ==
  Id : Inport
  Iq : Inport  Port=2
  Efd : Inport  Port=3
  Temp : Inport  Port=4
  Gain : Gain  Gain=Xd1 - Xls
  Gain1 : Gain  Gain=(Xd1 - Xd2)/(Xd1-Xls)^2
  Gain10 : Gain  Gain=Xq1 - Xls
  Gain11 : Gain  Gain=1/Tqo2
  Gain2 : Gain  Gain=Xd - Xd1
  Gain3 : Gain  Gain=1/Tdo1
  Gain4 : Gain  Gain=Xq1 - Xls
  Gain5 : Gain  Gain=(Xq1 - Xq2)/(Xq1 - Xls)^2
  Gain6 : Gain  Gain=Xq - Xq1
  Gain7 : Gain  Gain=1/Tqo1
  Gain8 : Gain  Gain=Xd1 - Xls
  Gain9 : Gain  Gain=1/Tdo2
  Integrator{,1..3} (4 alike) : Integrator
  Product{1..4} (4 alike) : Product
  Sum : Sum  Inputs=++-
  Sum1 : Sum  Inputs=+-
  Sum2 : Sum  Inputs=--+
  Sum3 : Sum  Inputs=+++
  Sum4 : Sum  Inputs=+-
  Sum5 : Sum  Inputs=-+
  Sum6 : Sum  Inputs=--+
  Sum7 : Sum  Inputs=---
  Eq1 : Outport
  Ed1 : Outport  Port=2
  Phi_1d : Outport  Port=3
  Phi_2q : Outport  Port=4
  wires:
  Efd/1 -> [Efd]
  Iq/1 -> [Iq]
  Id/1 -> [Id]
  Integrator3/1 -> Phi_2q/1, [Phi_2q]
  Sum7/1 -> Gain11/1
  [Ed1] -> Sum7/3
  [Phi_2q] -> Sum7/2
  Gain10/1 -> Sum7/1
  [Iq] -> Gain10/1
  Integrator2/1 -> Phi_1d/1, [Phi_1d]
  Sum6/1 -> Gain9/1
  [Eq1] -> Sum6/3
  [Phi_1d] -> Sum6/2
  Gain8/1 -> Sum6/1
  [Id] -> Gain8/1
  Sum5/1 -> Gain7/1
  Gain6/1 -> Sum5/2
  [Ed1] -> Sum5/1
  Sum4/1 -> Gain6/1
  Gain5/1 -> Sum4/2
  [Iq] -> Sum4/1
  Sum3/1 -> Gain5/1
  [Ed1] -> Sum3/3
  [Phi_2q] -> Sum3/2
  Gain4/1 -> Sum3/1
  [Iq] -> Gain4/1
  Integrator1/1 -> [Ed1], Ed1/1
  Sum2/1 -> Gain3/1
  [Efd] -> Sum2/3
  Gain2/1 -> Sum2/2
  [Eq1] -> Sum2/1
  Sum1/1 -> Gain2/1
  Gain1/1 -> Sum1/2
  [Id] -> Sum1/1
  Sum/1 -> Gain1/1
  [Eq1] -> Sum/3
  [Id] -> Gain/1
  Integrator/1 -> [Eq1], Eq1/1
  Gain/1 -> Sum/1
  [Phi_1d] -> Sum/2
  Temp/1 -> [R_temp_delta]
  [R_temp_delta] -> Product3/1
  Gain9/1 -> Product3/2
  Product3/1 -> Integrator2/1
  [R_temp_delta] -> Product1/1
  Gain11/1 -> Product1/2
  Product1/1 -> Integrator3/1
  [R_temp_delta] -> Product2/1
  Gain3/1 -> Product2/2
  Product2/1 -> Integrator/1
  [R_temp_delta] -> Product4/1
  Gain7/1 -> Product4/2
  Product4/1 -> Integrator1/1

== system Boeing787_debug/Electrical/Generation Unit Sync-Sync7/Generator/Electromagnetic Torque Output Power ==
  note: Torque from Damper Windings
  note: Torque from Field Winding
  Id : Inport
  Iq : Inport  Port=2
  Eq1 : Inport  Port=3
  Ed1 : Inport  Port=4
  Phi_1d : Inport  Port=5
  Phi_2q : Inport  Port=6
  Gain : Gain  Gain=(Xd2 - Xls)/(Xd1 - Xls)
  Gain1 : Gain  Gain=(Xq2 - Xls)/(Xq1 - Xls)
  Gain2 : Gain  Gain=(Xd1 - Xd2)/(Xd1-Xls)
  Gain3 : Gain  Gain=(Xq1 - Xq2)/(Xq1-Xls)
  Gain4 : Gain  Gain=(Xq2 - Xd2)
  Product{,1..4} (5 alike) : Product  RndMeth=Zero
  Sum : Sum
  Sum1 : Sum  Inputs=+-+
  Sum2 : Sum
  TE : Outport
  wires:
  Sum2/1 -> TE/1
  Sum1/1 -> Sum2/2
  Sum/1 -> Sum2/1
  Gain1/1 -> Sum/2
  Gain/1 -> Sum/1
  Gain4/1 -> Sum1/3
  Gain2/1 -> Sum1/1
  Gain3/1 -> Sum1/2
  Product4/1 -> Gain4/1
  [Iq] -> Product4/2
  [Id] -> Product4/1
  Product3/1 -> Gain3/1
  [Phi_2q] -> Product3/2
  [Id] -> Product3/1
  Product2/1 -> Gain2/1
  [Phi_1d] -> Product2/2
  [Iq] -> Product2/1
  Product1/1 -> Gain1/1
  [Id] -> Product1/2
  [Ed1] -> Product1/1
  Product/1 -> Gain/1
  [Iq] -> Product/2
  [Eq1] -> Product/1
  Iq/1 -> [Iq]
  Phi_2q/1 -> [Phi_2q]
  Phi_1d/1 -> [Phi_1d]
  Ed1/1 -> [Ed1]
  Eq1/1 -> [Eq1]
  Id/1 -> [Id]

== system Boeing787_debug/Electrical/Generation Unit Sync-Sync7/Generator/Generator Power Loss ==
  Ed : Inport
  Eq : Inport  Port=2
  Id : Inport  Port=3
  Iq : Inport  Port=4
  Te : Inport  Port=5
  w/ws : Inport  Port=6
  Bus Creator : BusCreator  Inputs=6
  Gain1 : Gain  Gain=SB
  Gain2 : Gain  Gain=SB
  Gain3 : Gain  Gain=SB
  Product : Product  RndMeth=Zero
  Product1 : Product  RndMeth=Zero
  Product2 : Product  RndMeth=Zero
  Sum1 : Sum  Inputs=-+
  Sum2 : Sum
  PE : Outport
  PM : Outport  Port=2
  PLOSS : Outport  Port=3
  m : Outport  Port=4
  wires:
  Gain3/1 -> PM/1
  Gain1/1 -> PE/1
  Gain2/1 -> PLOSS/1
  Bus Creator/1 -> m/1
  [nu] -> Bus Creator/6  "nu"
  [Te] -> Bus Creator/5  "Te"
  [Iq] -> Bus Creator/4  "Iq"
  [Eq] -> Bus Creator/3  "Vq"
  [Id] -> Bus Creator/2  "Id"
  [Ed] -> Bus Creator/1  "Vd"
  Sum1/1 -> Gain2/1
  Product2/1 -> Gain3/1, Sum1/2
  Sum2/1 -> Gain1/1, Sum1/1
  Product1/1 -> Sum2/2
  Product/1 -> Sum2/1
  [nu] -> Product2/2
  [Te] -> Product2/1
  [Iq] -> Product1/2
  [Eq] -> Product1/1
  [Id] -> Product/2
  [Ed] -> Product/1
  w/ws/1 -> [nu]
  Te/1 -> [Te]
  Iq/1 -> [Iq]
  Id/1 -> [Id]
  Eq/1 -> [Eq]
  Ed/1 -> [Ed]

== system Boeing787_debug/Electrical/Generation Unit Sync-Sync7/Generator/Stator Voltage ==
  Id : Inport
  Iq : Inport  Port=2
  Eq1 : Inport  Port=3
  Ed1 : Inport  Port=4
  Phi_1d : Inport  Port=5
  Phi_2q : Inport  Port=6
  w/ws : Inport  Port=7
  Temp : Inport  Port=8
  Gain : Gain  Gain=(Xq2 - Xls)/(Xq1 - Xls)
  Gain1 : Gain  Gain=(Xq1 - Xq2)/(Xq1 - Xls)
  Gain2 : Gain  Gain=(Xq2 - Xd2)
  Gain3 : Gain  Gain=(Xd2 - Xls)/(Xd1 - Xls)
  Gain4 : Gain  Gain=(Xd1 - Xd2)/(Xd1 - Xls)
  Gain5 : Gain  Gain=Rs
  Gain6 : Gain  Gain=Xd2
  Gain7 : Gain  Gain=Rs
  Gain8 : Gain  Gain=Xd2
  Product{,1..3,5} (5 alike) : Product  RndMeth=Zero
  Product4 : Product
  Sum : Sum
  Sum1 : Sum  Inputs=+-+
  Sum2 : Sum  Inputs=--+
  Sum3 : Sum  Inputs=-++
  Ed : Outport
  Eq : Outport  Port=2
  wires:
  Gain7/1 -> Sum2/2
  Product3/1 -> Sum2/1
  Sum2/1 -> Eq/1  "Vq"
  Sum3/1 -> Ed/1  "Vd"
  Product2/1 -> Sum3/3
  Product1/1 -> Sum3/2
  Gain8/1 -> Product3/1
  Gain6/1 -> Product2/2
  Id/1 -> Gain8/1, Gain5/1
  Product/1 -> Sum2/3
  w/ws/1 -> Product2/1, Product3/2, Product/2, Product1/2
  Sum1/1 -> Product1/1
  Sum/1 -> Product/1
  Gain1/1 -> Sum1/2
  Gain/1 -> Sum1/1
  Gain3/1 -> Sum/1
  Gain4/1 -> Sum/2
  Phi_1d/1 -> Gain4/1
  Eq1/1 -> Gain3/1
  Phi_2q/1 -> Gain1/1
  Ed1/1 -> Gain/1
  Gain2/1 -> Sum1/3
  Temp/1 -> Product5/1, Product4/2
  Gain5/1 -> Product4/1
  Product4/1 -> Sum3/1
  Product5/1 -> Gain7/1
  Iq/1 -> Gain2/1, Product5/2, Gain6/1

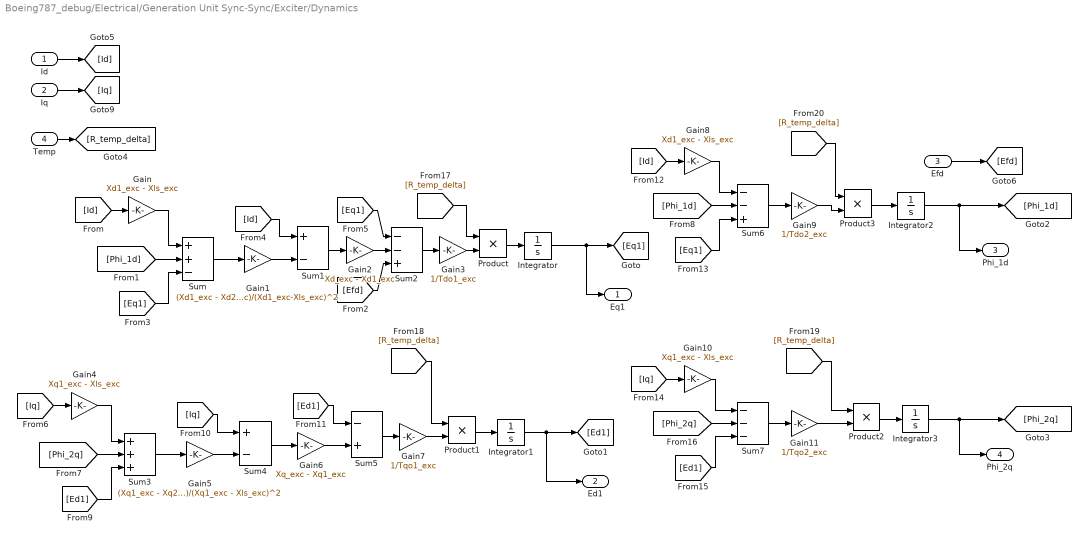
== system Boeing787_debug/Electrical/Generation Unit Sync-Sync/Exciter/Dynamics ==
  Id : Inport
  Iq : Inport  Port=2
  Efd : Inport  Port=3
  Temp : Inport  Port=4
  Gain : Gain  Gain=Xd1_exc - Xls_exc
  Gain1 : Gain  Gain=(Xd1_exc - Xd2_exc)/(Xd1_exc-Xls_exc)^2
  Gain10 : Gain  Gain=Xq1_exc - Xls_exc
  Gain11 : Gain  Gain=1/Tqo2_exc
  Gain2 : Gain  Gain=Xd_exc - Xd1_exc
  Gain3 : Gain  Gain=1/Tdo1_exc
  Gain4 : Gain  Gain=Xq1_exc - Xls_exc
  Gain5 : Gain  Gain=(Xq1_exc - Xq2_exc)/(Xq1_exc - Xls_exc)^2
  Gain6 : Gain  Gain=Xq_exc - Xq1_exc
  Gain7 : Gain  Gain=1/Tqo1_exc
  Gain8 : Gain  Gain=Xd1_exc - Xls_exc
  Gain9 : Gain  Gain=1/Tdo2_exc
  Integrator{,1..3} (4 alike) : Integrator
  Product{,1..3} (4 alike) : Product
  Sum : Sum  Inputs=++-
  Sum1 : Sum  Inputs=+-
  Sum2 : Sum  Inputs=--+
  Sum3 : Sum  Inputs=+++
  Sum4 : Sum  Inputs=+-
  Sum5 : Sum  Inputs=-+
  Sum6 : Sum  Inputs=--+
  Sum7 : Sum  Inputs=---
  Eq1 : Outport
  Ed1 : Outport  Port=2
  Phi_1d : Outport  Port=3
  Phi_2q : Outport  Port=4
  wires:
  Product3/1 -> Integrator2/1
  Gain9/1 -> Product3/2
  [R_temp_delta] -> Product3/1
  Product2/1 -> Integrator3/1
  Gain11/1 -> Product2/2
  [R_temp_delta] -> Product2/1
  Product1/1 -> Integrator1/1
  Gain7/1 -> Product1/2
  [R_temp_delta] -> Product1/1
  [R_temp_delta] -> Product/1
  Product/1 -> Integrator/1
  Gain3/1 -> Product/2
  Temp/1 -> [R_temp_delta]
  Efd/1 -> [Efd]
  Iq/1 -> [Iq]
  Id/1 -> [Id]
  Integrator3/1 -> Phi_2q/1, [Phi_2q]
  Sum7/1 -> Gain11/1
  [Ed1] -> Sum7/3
  [Phi_2q] -> Sum7/2
  Gain10/1 -> Sum7/1
  [Iq] -> Gain10/1
  Integrator2/1 -> Phi_1d/1, [Phi_1d]
  Sum6/1 -> Gain9/1
  [Eq1] -> Sum6/3
  [Phi_1d] -> Sum6/2
  Gain8/1 -> Sum6/1
  [Id] -> Gain8/1
  Sum5/1 -> Gain7/1
  Gain6/1 -> Sum5/2
  [Ed1] -> Sum5/1
  Sum4/1 -> Gain6/1
  Gain5/1 -> Sum4/2
  [Iq] -> Sum4/1
  Sum3/1 -> Gain5/1
  [Ed1] -> Sum3/3
  [Phi_2q] -> Sum3/2
  Gain4/1 -> Sum3/1
  [Iq] -> Gain4/1
  Integrator1/1 -> [Ed1], Ed1/1
  Sum2/1 -> Gain3/1
  [Efd] -> Sum2/3
  Gain2/1 -> Sum2/2
  [Eq1] -> Sum2/1
  Sum1/1 -> Gain2/1
  Gain1/1 -> Sum1/2
  [Id] -> Sum1/1
  Sum/1 -> Gain1/1
  [Eq1] -> Sum/3
  [Phi_1d] -> Sum/2
  Gain/1 -> Sum/1
  [Id] -> Gain/1
  Integrator/1 -> [Eq1], Eq1/1

== system Boeing787_debug/Electrical/Generation Unit Sync-Sync/Exciter/Electromagnetic Torque Output Power ==
  note: Torque from Damper Windings
  note: Torque from Field Winding
  Id : Inport
  Iq : Inport  Port=2
  Eq1 : Inport  Port=3
  Ed1 : Inport  Port=4
  Phi_1d : Inport  Port=5
  Phi_2q : Inport  Port=6
  Gain : Gain  Gain=(Xd2_exc - Xls_exc)/(Xd1_exc - Xls_exc)
  Gain1 : Gain  Gain=(Xq2_exc - Xls_exc)/(Xq1_exc - Xls_exc)
  Gain2 : Gain  Gain=(Xd1_exc - Xd2_exc)/(Xd1_exc-Xls_exc)
  Gain3 : Gain  Gain=(Xq1_exc - Xq2_exc)/(Xq1_exc-Xls_exc)
  Gain4 : Gain  Gain=(Xq2_exc - Xd2_exc)
  Product{,1..4} (5 alike) : Product  RndMeth=Zero
  Sum : Sum
  Sum1 : Sum  Inputs=+-+
  Sum2 : Sum
  TE : Outport
  wires:
  Sum2/1 -> TE/1
  Sum1/1 -> Sum2/2
  Sum/1 -> Sum2/1
  Gain1/1 -> Sum/2
  Gain/1 -> Sum/1
  Gain4/1 -> Sum1/3
  Gain2/1 -> Sum1/1
  Gain3/1 -> Sum1/2
  Product4/1 -> Gain4/1
  [Iq] -> Product4/2
  [Id] -> Product4/1
  Product3/1 -> Gain3/1
  [Phi_2q] -> Product3/2
  [Id] -> Product3/1
  Product2/1 -> Gain2/1
  [Phi_1d] -> Product2/2
  [Iq] -> Product2/1
  Product1/1 -> Gain1/1
  [Id] -> Product1/2
  [Ed1] -> Product1/1
  Product/1 -> Gain/1
  [Iq] -> Product/2
  [Eq1] -> Product/1
  Iq/1 -> [Iq]
  Phi_2q/1 -> [Phi_2q]
  Phi_1d/1 -> [Phi_1d]
  Ed1/1 -> [Ed1]
  Eq1/1 -> [Eq1]
  Id/1 -> [Id]

== system Boeing787_debug/Electrical/Generation Unit Sync-Sync/Exciter/Generator Power Loss ==
  Ed : Inport
  Eq : Inport  Port=2
  Id : Inport  Port=3
  Iq : Inport  Port=4
  Te : Inport  Port=5
  w/ws : Inport  Port=6
  Bus Creator : BusCreator  Inputs=6
  Gain1 : Gain  Gain=SB_exc
  Gain2 : Gain  Gain=SB_exc
  Gain3 : Gain  Gain=SB_exc
  Product : Product  RndMeth=Zero
  Product1 : Product  RndMeth=Zero
  Product2 : Product  RndMeth=Zero
  Sum1 : Sum  Inputs=-+
  Sum2 : Sum
  PE : Outport
  PM : Outport  Port=2
  PLOSS : Outport  Port=3
  m : Outport  Port=4
  wires:
  Gain3/1 -> PM/1
  Gain1/1 -> PE/1
  Gain2/1 -> PLOSS/1
  Bus Creator/1 -> m/1
  [nu] -> Bus Creator/6  "nu"
  [Te] -> Bus Creator/5  "Te"
  [Iq] -> Bus Creator/4  "Iq"
  [Eq] -> Bus Creator/3  "Vq"
  [Id] -> Bus Creator/2  "Id"
  [Ed] -> Bus Creator/1  "Vd"
  Sum1/1 -> Gain2/1
  Product2/1 -> Gain3/1, Sum1/2
  Sum2/1 -> Gain1/1, Sum1/1
  Product1/1 -> Sum2/2
  Product/1 -> Sum2/1
  [nu] -> Product2/2
  [Te] -> Product2/1
  [Iq] -> Product1/2
  [Eq] -> Product1/1
  [Id] -> Product/2
  [Ed] -> Product/1
  w/ws/1 -> [nu]
  Te/1 -> [Te]
  Iq/1 -> [Iq]
  Id/1 -> [Id]
  Eq/1 -> [Eq]
  Ed/1 -> [Ed]

== system Boeing787_debug/Electrical/Generation Unit Sync-Sync/Exciter/Stator Voltage ==
  Id : Inport
  Iq : Inport  Port=2
  Eq1 : Inport  Port=3
  Ed1 : Inport  Port=4
  Phi_1d : Inport  Port=5
  Phi_2q : Inport  Port=6
  w/ws : Inport  Port=7
  Temp : Inport  Port=8
  Gain : Gain  Gain=(Xq2_exc - Xls_exc)/(Xq1_exc - Xls_exc)
  Gain1 : Gain  Gain=(Xq1_exc - Xq2_exc)/(Xq1_exc - Xls_exc)
  Gain2 : Gain  Gain=(Xq2_exc - Xd2_exc)
  Gain3 : Gain  Gain=(Xd2_exc - Xls_exc)/(Xd1_exc - Xls_exc)
  Gain4 : Gain  Gain=(Xd1_exc - Xd2_exc)/(Xd1_exc - Xls_exc)
  Gain5 : Gain  Gain=Rs_exc
  Gain6 : Gain  Gain=Xd2+XTL
  Gain7 : Gain  Gain=Rs_exc+RTL_exc
  Gain8 : Gain  Gain=Xd2_exc+XTL_exc
  Product{,1..3,5} (5 alike) : Product  RndMeth=Zero
  Product4 : Product
  Sum : Sum
  Sum1 : Sum  Inputs=+-+
  Sum2 : Sum  Inputs=--+
  Sum3 : Sum  Inputs=-++
  Ed : Outport
  Eq : Outport  Port=2
  wires:
  Product5/1 -> Gain7/1
  Temp/1 -> Product4/2, Product5/1
  Gain5/1 -> Product4/1
  Product4/1 -> Sum3/1
  Gain7/1 -> Sum2/2
  Product3/1 -> Sum2/1
  Sum2/1 -> Eq/1  "Vq"
  Sum3/1 -> Ed/1  "Vd"
  Product2/1 -> Sum3/3
  Gain2/1 -> Sum1/3
  Product1/1 -> Sum3/2
  Gain8/1 -> Product3/1
  Gain6/1 -> Product2/2
  Id/1 -> Gain8/1, Gain5/1
  Product/1 -> Sum2/3
  w/ws/1 -> Product2/1, Product3/2, Product/2, Product1/2
  Sum1/1 -> Product1/1
  Sum/1 -> Product/1
  Gain1/1 -> Sum1/2
  Gain/1 -> Sum1/1
  Gain3/1 -> Sum/1
  Gain4/1 -> Sum/2
  Phi_1d/1 -> Gain4/1
  Eq1/1 -> Gain3/1
  Iq/1 -> Gain2/1, Gain6/1, Product5/2
  Phi_2q/1 -> Gain1/1
  Ed1/1 -> Gain/1

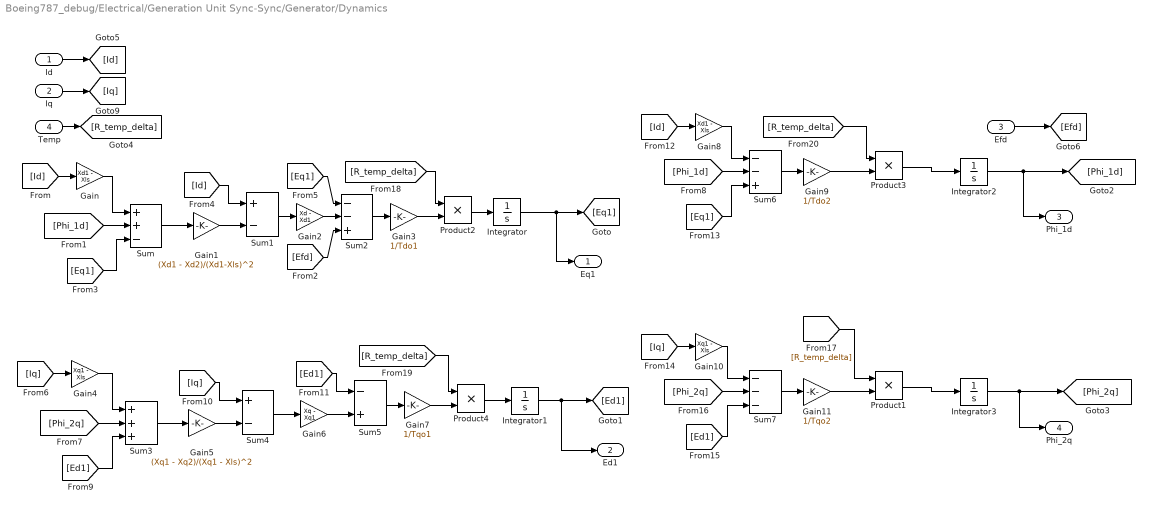
== system Boeing787_debug/Electrical/Generation Unit Sync-Sync/Generator/Dynamics ==
  Id : Inport
  Iq : Inport  Port=2
  Efd : Inport  Port=3
  Temp : Inport  Port=4
  Gain : Gain  Gain=Xd1 - Xls
  Gain1 : Gain  Gain=(Xd1 - Xd2)/(Xd1-Xls)^2
  Gain10 : Gain  Gain=Xq1 - Xls
  Gain11 : Gain  Gain=1/Tqo2
  Gain2 : Gain  Gain=Xd - Xd1
  Gain3 : Gain  Gain=1/Tdo1
  Gain4 : Gain  Gain=Xq1 - Xls
  Gain5 : Gain  Gain=(Xq1 - Xq2)/(Xq1 - Xls)^2
  Gain6 : Gain  Gain=Xq - Xq1
  Gain7 : Gain  Gain=1/Tqo1
  Gain8 : Gain  Gain=Xd1 - Xls
  Gain9 : Gain  Gain=1/Tdo2
  Integrator{,1..3} (4 alike) : Integrator
  Product{1..4} (4 alike) : Product
  Sum : Sum  Inputs=++-
  Sum1 : Sum  Inputs=+-
  Sum2 : Sum  Inputs=--+
  Sum3 : Sum  Inputs=+++
  Sum4 : Sum  Inputs=+-
  Sum5 : Sum  Inputs=-+
  Sum6 : Sum  Inputs=--+
  Sum7 : Sum  Inputs=---
  Eq1 : Outport
  Ed1 : Outport  Port=2
  Phi_1d : Outport  Port=3
  Phi_2q : Outport  Port=4
  wires:
  Product4/1 -> Integrator1/1
  Gain7/1 -> Product4/2
  [R_temp_delta] -> Product4/1
  Product2/1 -> Integrator/1
  Gain3/1 -> Product2/2
  [R_temp_delta] -> Product2/1
  Product1/1 -> Integrator3/1
  Gain11/1 -> Product1/2
  [R_temp_delta] -> Product1/1
  Product3/1 -> Integrator2/1
  Gain9/1 -> Product3/2
  [R_temp_delta] -> Product3/1
  Temp/1 -> [R_temp_delta]
  [Phi_1d] -> Sum/2
  Gain/1 -> Sum/1
  Integrator/1 -> Eq1/1, [Eq1]
  [Id] -> Gain/1
  [Eq1] -> Sum/3
  Sum/1 -> Gain1/1
  [Id] -> Sum1/1
  Gain1/1 -> Sum1/2
  Sum1/1 -> Gain2/1
  [Eq1] -> Sum2/1
  Gain2/1 -> Sum2/2
  [Efd] -> Sum2/3
  Sum2/1 -> Gain3/1
  Integrator1/1 -> Ed1/1, [Ed1]
  [Iq] -> Gain4/1
  Gain4/1 -> Sum3/1
  [Phi_2q] -> Sum3/2
  [Ed1] -> Sum3/3
  Sum3/1 -> Gain5/1
  [Iq] -> Sum4/1
  Gain5/1 -> Sum4/2
  Sum4/1 -> Gain6/1
  [Ed1] -> Sum5/1
  Gain6/1 -> Sum5/2
  Sum5/1 -> Gain7/1
  [Id] -> Gain8/1
  Gain8/1 -> Sum6/1
  [Phi_1d] -> Sum6/2
  [Eq1] -> Sum6/3
  Sum6/1 -> Gain9/1
  Integrator2/1 -> [Phi_1d], Phi_1d/1
  [Iq] -> Gain10/1
  Gain10/1 -> Sum7/1
  [Phi_2q] -> Sum7/2
  [Ed1] -> Sum7/3
  Sum7/1 -> Gain11/1
  Integrator3/1 -> [Phi_2q], Phi_2q/1
  Id/1 -> [Id]
  Iq/1 -> [Iq]
  Efd/1 -> [Efd]

== system Boeing787_debug/Electrical/Generation Unit Sync-Sync/Generator/Electromagnetic Torque Output Power ==
  note: Torque from Field Winding
  note: Torque from Damper Windings
  Id : Inport
  Iq : Inport  Port=2
  Eq1 : Inport  Port=3
  Ed1 : Inport  Port=4
  Phi_1d : Inport  Port=5
  Phi_2q : Inport  Port=6
  Gain : Gain  Gain=(Xd2 - Xls)/(Xd1 - Xls)
  Gain1 : Gain  Gain=(Xq2 - Xls)/(Xq1 - Xls)
  Gain2 : Gain  Gain=(Xd1 - Xd2)/(Xd1-Xls)
  Gain3 : Gain  Gain=(Xq1 - Xq2)/(Xq1-Xls)
  Gain4 : Gain  Gain=(Xq2 - Xd2)
  Product{,1..4} (5 alike) : Product  RndMeth=Zero
  Scope{,1..4} (5 alike) : Scope
      Scope settings: YMin=-0.00574  YMax=0.05167  SaveName=ScopeData2
      Scope1 settings: YMin=-0.04047  YMax=0.36422  SaveName=ScopeData3
      Scope2 settings: YMin=-0.001  YMax=0.00903  SaveName=ScopeData4
      Scope3 settings: YMin=-0.0032  YMax=0.00036  SaveName=ScopeData5
      Scope4 settings: YMin=0.06667  YMax=0.26667  SaveName=ScopeData6
  Sum : Sum
  Sum1 : Sum  Inputs=+-+
  Sum2 : Sum
  TE : Outport
  wires:
  Id/1 -> [Id]
  Eq1/1 -> [Eq1]
  Ed1/1 -> [Ed1]
  Phi_1d/1 -> [Phi_1d]
  Phi_2q/1 -> [Phi_2q]
  Iq/1 -> [Iq]
  [Iq] -> Scope4/1, Product/2
  Product/1 -> Scope3/1, Gain/1
  [Ed1] -> Product1/1
  [Id] -> Product1/2
  Product1/1 -> Gain1/1
  [Iq] -> Product2/1
  [Phi_1d] -> Product2/2
  Product2/1 -> Gain2/1
  [Id] -> Product3/1
  [Phi_2q] -> Product3/2
  Product3/1 -> Gain3/1
  [Id] -> Product4/1
  [Iq] -> Product4/2
  Product4/1 -> Gain4/1
  Gain3/1 -> Sum1/2
  Gain2/1 -> Sum1/1, Scope2/1
  Gain4/1 -> Sum1/3
  Gain/1 -> Scope/1, Sum/1
  Gain1/1 -> Sum/2
  Sum/1 -> Sum2/1
  Sum1/1 -> Sum2/2
  Sum2/1 -> TE/1
  [Eq1] -> Scope1/1, Product/1

== system Boeing787_debug/Electrical/Generation Unit Sync-Sync/Generator/Generator Power Loss ==
  Ed : Inport
  Eq : Inport  Port=2
  Id : Inport  Port=3
  Iq : Inport  Port=4
  Te : Inport  Port=5
  w/ws : Inport  Port=6
  Bus Creator : BusCreator  Inputs=6
  Gain1 : Gain  Gain=SB
  Gain2 : Gain  Gain=SB
  Gain3 : Gain  Gain=SB
  Product : Product  RndMeth=Zero
  Product1 : Product  RndMeth=Zero
  Product2 : Product  RndMeth=Zero
  Sum1 : Sum  Inputs=-+
  Sum2 : Sum
  PE : Outport
  PM : Outport  Port=2
  PLOSS : Outport  Port=3
  m : Outport  Port=4
  wires:
  Ed/1 -> [Ed]
  Eq/1 -> [Eq]
  Id/1 -> [Id]
  Iq/1 -> [Iq]
  Te/1 -> [Te]
  w/ws/1 -> [nu]
  [Ed] -> Product/1
  [Id] -> Product/2
  [Eq] -> Product1/1
  [Iq] -> Product1/2
  [Te] -> Product2/1
  [nu] -> Product2/2
  Product/1 -> Sum2/1
  Product1/1 -> Sum2/2
  Sum2/1 -> Sum1/1, Gain1/1
  Product2/1 -> Sum1/2, Gain3/1
  Sum1/1 -> Gain2/1
  [Ed] -> Bus Creator/1  "Vd"
  [Id] -> Bus Creator/2  "Id"
  [Eq] -> Bus Creator/3  "Vq"
  [Iq] -> Bus Creator/4  "Iq"
  [Te] -> Bus Creator/5  "Te"
  [nu] -> Bus Creator/6  "nu"
  Bus Creator/1 -> m/1
  Gain2/1 -> PLOSS/1
  Gain1/1 -> PE/1
  Gain3/1 -> PM/1

== system Boeing787_debug/Electrical/Generation Unit Sync-Sync/Generator/Stator Voltage ==
  Id : Inport
  Iq : Inport  Port=2
  Eq1 : Inport  Port=3
  Ed1 : Inport  Port=4
  Phi_1d : Inport  Port=5
  Phi_2q : Inport  Port=6
  w/ws : Inport  Port=7
  Temp : Inport  Port=8
  Gain : Gain  Gain=(Xq2 - Xls)/(Xq1 - Xls)
  Gain1 : Gain  Gain=(Xq1 - Xq2)/(Xq1 - Xls)
  Gain2 : Gain  Gain=(Xq2 - Xd2)
  Gain3 : Gain  Gain=(Xd2 - Xls)/(Xd1 - Xls)
  Gain4 : Gain  Gain=(Xd1 - Xd2)/(Xd1 - Xls)
  Gain5 : Gain  Gain=Rs
  Gain6 : Gain  Gain=Xd2
  Gain7 : Gain  Gain=Rs
  Gain8 : Gain  Gain=Xd2
  Product{,1..3,5} (5 alike) : Product  RndMeth=Zero
  Product4 : Product
  Sum : Sum
  Sum1 : Sum  Inputs=+-+
  Sum2 : Sum  Inputs=--+
  Sum3 : Sum  Inputs=-++
  Ed : Outport
  Eq : Outport  Port=2
  wires:
  Iq/1 -> Gain6/1, Product5/2, Gain2/1
  Product5/1 -> Gain7/1
  Product4/1 -> Sum3/1
  Gain5/1 -> Product4/1
  Temp/1 -> Product4/2, Product5/1
  Gain2/1 -> Sum1/3
  Ed1/1 -> Gain/1
  Phi_2q/1 -> Gain1/1
  Eq1/1 -> Gain3/1
  Phi_1d/1 -> Gain4/1
  Gain4/1 -> Sum/2
  Gain3/1 -> Sum/1
  Gain/1 -> Sum1/1
  Gain1/1 -> Sum1/2
  Sum/1 -> Product/1
  Sum1/1 -> Product1/1
  w/ws/1 -> Product1/2, Product/2, Product3/2, Product2/1
  Product/1 -> Sum2/3
  Id/1 -> Gain5/1, Gain8/1
  Gain6/1 -> Product2/2
  Gain8/1 -> Product3/1
  Product1/1 -> Sum3/2
  Product2/1 -> Sum3/3
  Sum3/1 -> Ed/1  "Vd"
  Sum2/1 -> Eq/1  "Vq"
  Product3/1 -> Sum2/1
  Gain7/1 -> Sum2/2
